simulink model "DepthSemanticSegmentation"  (R2021a)
settings: Solver=VariableStepAuto  StartTime=0.0  StopTime=10.0  RelTol=1e-3
libraries: visionsinks x3, sim3dcameralib x1, sim3dlib x1, uavsim3dlib x1, simulink x1
settings Model: Creator=student  LastModifiedBy=student

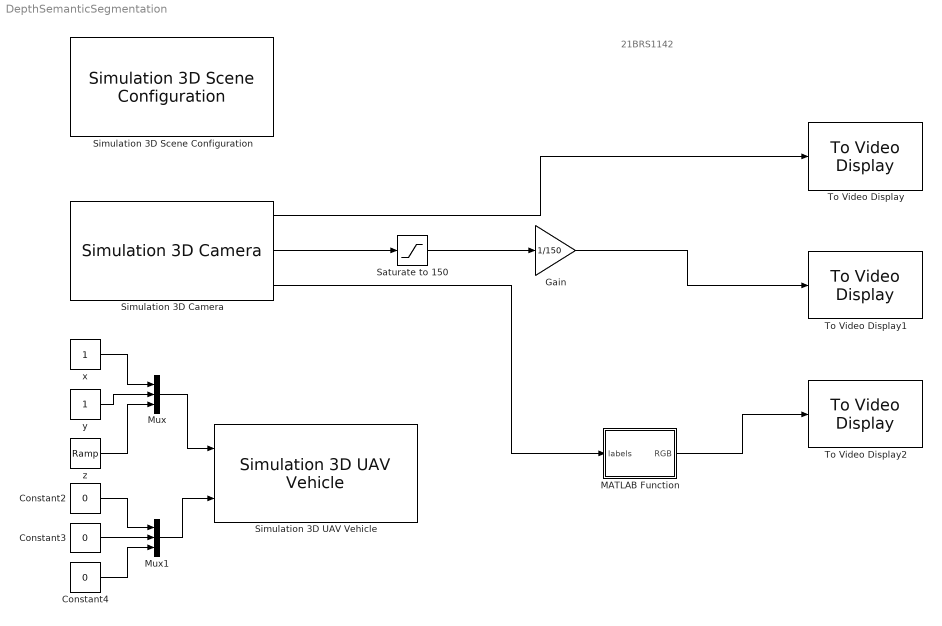
== system DepthSemanticSegmentation ==
  note: 21BRS1142
  Constant2 : Constant  Value=0
  Constant3 : Constant  Value=0
  Constant4 : Constant  Value=0
  Gain : Gain  Gain=1/150
  MATLAB Function : MATLAB Function  TreatAsAtomicUnit=on
  Mux : Mux  Inputs=3
  Mux1 : Mux  Inputs=3
  Saturate to 150 : Saturate  UpperLimit=150
  Simulation 3D Camera : sim3dcameralib/Simulation 3D Camera  Priority=1  sensorTag=Sim3dSensor1  sensorId=1  sensorName=Sim3dSensor1  vehTagList={'Scene Origin';'SimulinkVehicle1'}  vehTag=Scene Origin  mountLoc=Origin  offsetFlag=on  tmountOffset=[0, 0, 0]  rmountOffset=[0, 0, 0]  FocalLength=[1109, 1109]  OpticalCenter=[640, 360]  ImageSize=[720, 1280]  RadialDistortion=[0, 0]  TangentialDistortion=[0, 0]  SensorSkew=0  DepthOutportEnabled=on  SemanticOutportEnabled=on  TransformOutportEnabled=off  SampleTime=-1  mountPoint=[0 0 0]  mountOrientation=[0 0 0]  aMode=4  ID=1
      settings: SourceProductBaseCode=DR,UV,VE
  Simulation 3D Scene Configuration : sim3dlib/Simulation 3D Scene Configuration  Priority=0  ProjectFormat=Default Scenes  SceneDesc=US city block  ProjectName=C:\Program Files\MATLAB\R2021a\toolbox\shared\sim3d_projects\automotive_project\UE4\WindowsNoEditor\VehicleSimulation.exe  ScenePath=/Game/Maps/USCityBlock  vehTagList={'Scene Origin';'SimulinkVehicle1'}  vehTag=Scene Origin  OpVisEn=off  Ts=1/60  EnableWindow=on  EnableWeather=off  SunAltitude=40.0  SunAzimuth=90  clouds=10  wind=1  fog=0  rain=0  sensorTag=MainCamera1  sensorId=1  sensorName=MainCamera1  mountLoc=Origin  offsetFlag=off  tmountOffset=[0, 0, 0]  rmountOffset=[0, 0, 0]  HorizontalResolution=1280  VerticalResolution=720  HorizontalFOV=60  mountPoint=[0 0 0]  mountOrientation=[0 0 0]  aMode=4  ID=1
      settings: SourceProductBaseCode=DR,UV,VE
  Simulation 3D UAV Vehicle : uavsim3dlib/Simulation 3D UAV Vehicle  Priority=-1  Mesh=Quadrotor  Color=Black  ActorName=SimulinkVehicle1  InitialTranslation=[0 0 0]  InitialRotation=[0 0 0]  SampleTime=-1  ActorType=SimulinkVehicle  ID=1  aMode=4  ActorTag=SimulinkVehicle1
      settings: SourceProductBaseCode=UV
  To Video Display : visionsinks/To Video Display  windowSizeMode=Normal  openAtMdlStart=on  fullScreen=off  videoWindowX=536805376  videoWindowY=536805376  saveWindowSize=off  videoWindowWidth=2147483647  videoWindowHeight=2147483647  inputColorFormat=RGB  inputType=Obsolete  imagePorts=One multidimensional signal  OutputDevice=On-screen video monitor  dataOrg=Column-major  isWindowOpen=off
  To Video Display1 : visionsinks/To Video Display  windowSizeMode=Normal  openAtMdlStart=on  fullScreen=off  videoWindowX=536805376  videoWindowY=536805376  saveWindowSize=off  videoWindowWidth=2147483647  videoWindowHeight=2147483647  inputColorFormat=RGB  inputType=Obsolete  imagePorts=One multidimensional signal  OutputDevice=On-screen video monitor  dataOrg=Column-major  isWindowOpen=off
  To Video Display2 : visionsinks/To Video Display  windowSizeMode=Normal  openAtMdlStart=on  fullScreen=off  videoWindowX=536805376  videoWindowY=536805376  saveWindowSize=off  videoWindowWidth=2147483647  videoWindowHeight=2147483647  inputColorFormat=RGB  inputType=Obsolete  imagePorts=One multidimensional signal  OutputDevice=On-screen video monitor  dataOrg=Column-major  isWindowOpen=off
  x : Constant
  y : Constant
  z : simulink/Sources/Ramp  slope=1  start=0  InitialOutput=0
  wires:
  x/1 -> Mux/1
  y/1 -> Mux/2
  z/1 -> Mux/3
  Constant2/1 -> Mux1/1
  Constant3/1 -> Mux1/2
  Constant4/1 -> Mux1/3
  Mux1/1 -> Simulation 3D UAV Vehicle/2
  Mux/1 -> Simulation 3D UAV Vehicle/1
  Simulation 3D Camera/3 -> MATLAB Function/1(labels)
  Simulation 3D Camera/1 -> To Video Display/1
  Simulation 3D Camera/2 -> Saturate to 150/1
  Saturate to 150/1 -> Gain/1
  Gain/1 -> To Video Display1/1
  MATLAB Function/1(RGB) -> To Video Display2/1

== matlab function DepthSemanticSegmentation/MATLAB Function ==
  data: labels input; RGB output
function RGB = uavlabel2rgb(labels)

coder.extrinsic('label2rgb');
RGB = coder.nullcopy(zeros(size(labels, 1), size(labels, 2), 3, class(labels)));
cmap = sim3dColormap;
RGB = label2rgb(labels, cmap);

end 

function cmap = sim3dColormap
% Define colormap for object labels used in 3D simulation environment.
cmap = [
    150 90 150 % Label 1: Building
    0 0 0 % Label 2: Not used
    72 0 90 % Label 3: Other
    0 0 0 % Label 4: Not used
    192 192 192 % Label 5: Pole
    128 0 128 % Label 6: Lane marking
    128 64 128 % Label 7: Roads
    60 40 222 % Label 8: Sidewalk
    120 128 100 % Label 9: Vegetation
    64 0 128 % Label 10: Vehicle
    0 0 0 % Label 11: Not used
    192 128 128 % Label 12: Generic traffic signs
    192 128 128 % Label 13: Stop sign
    192 128 128 % Label 14: Yield sign
    192 128 128 % Label 15: Speed limit sign
    192 128 128 % Label 16: Weight limit sign
    0 0 0 % Label 17: Not used
    0 0 0 % Label 18: Not used
    192 128 128 % Label 19: Left and right arrow warning sign
    192 128 128 % Label 20: Left chevron warning sign
    192 128 128 % Label 21: Right chevron warning sign
    0 0 0 % Label 22: Not used
    192 128 128 % Label 23: Right one-way sign
    0 0 0 % Label 24: Not used
    192 128 128 % Label 25: School bus only sign
    0 0 0 % Label 26: Not used
    0 0 0 % Label 27: Not used
    0 0 0 % Label 28: Not used
    0 0 0 % Label 29: Not used
    0 0 0 % Label 30: Not used
    0 0 0 % Label 31: Not used
    0 0 0 % Label 32: Not used
    0 0 0 % Label 33: Not used
    0 0 0 % Label 34: Not used
    0 0 0 % Label 35: Not used
    0 0 0 % Label 36: Not used
    0 0 0 % Label 37: Not used
    0 0 0 % Label 38: Not used
    192 128 128 % Label 39: Crosswalk sign
    0 0 0 % Label 40: Not used
    192 128 128 % Label 41: Traffic signal
    192 128 128 % Label 42: Curve right warning sign
    192 128 128 % Label 43: Curve left warning sign
    192 128 128 % Label 44: Up right arrow warning sign
    0 0 0 % Label 45: Not used
    0 0 0 % Label 46: Not used
    0 0 0 % Label 47: Not used
    192 128 128 % Label 48: Railroad crossing sign
    192 128 128 % Label 49: Street sign
    192 128 128 % Label 50: Roundabout warning sign
    192 128 128 % Label 51: Fire hydrant
    192 128 128 % Label 52: Exit sign
    192 128 128 % Label 53: Bike lane sign
    0 0 0 % Label 54: Not used
    0 0 0 % Label 55: Not used
    0 0 0 % Label 56: Not used
    128 128 128 % Label 57: Sky
    60 40 222 % Label 58: Curb
    60 40 222 % Label 59: Flyover ramp
    60 40 222 % Label 60: Road guard rail
    0 0 0 % Label 61: Not used
    0 0 0 % Label 62: Not used
    0 0 0 % Label 63: Not used
    0 0 0 % Label 64: Not used
    0 0 0 % Label 65: Not used
    0 0 0 % Label 66: Not used
    240 150 25 % Label 67: Deer
    0 0 0 % Label 68: Not used
    0 0 0 % Label 69: Not used
    0 0 0 % Label 70: Not used
    150 50 15 % Label 71: Barricade
    0 128 192 % Label 72: Motorcycle
];
% Normalize colormap to the range [0, 1].
cmap = cmap ./ 255;
end
